simulink model "mvdc_vehicle_dynamics_control"  (R2018b)
settings: configuration reference "Active" (kept outside this file)
undefined symbols (not defined in the file): IC_TUMModeControl, tS
libraries: simulink x1
settings Model: DataDictionary=mvdc_vehicle_dynamics_control.sldd  Creator=wischnewski  LastModifiedBy=ga25xiw

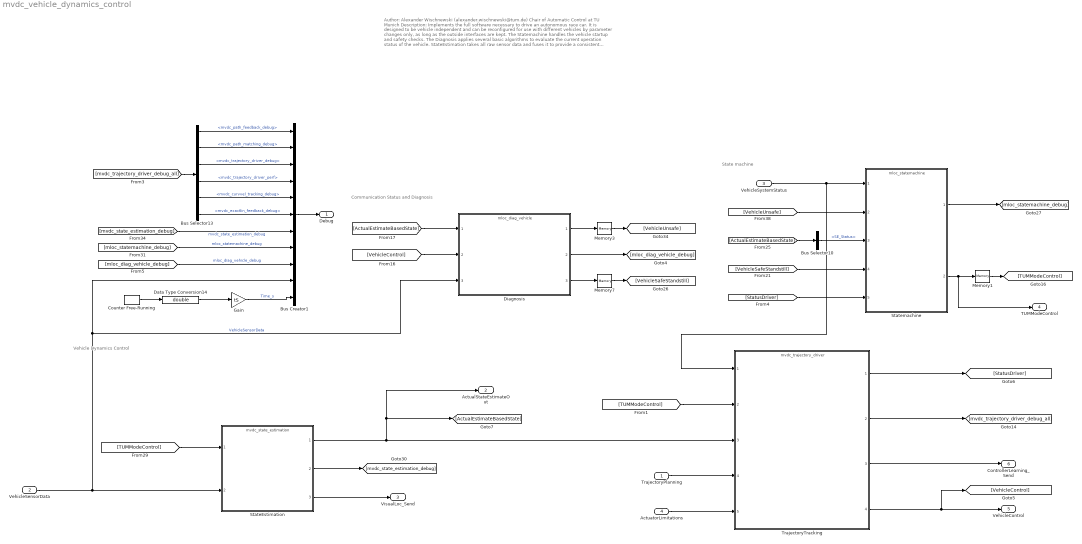
== system mvdc_vehicle_dynamics_control ==
  note: Communication Status and Diagnosis
  note: Vehicle Dynamics Control
  note: State machine
  note: Author: Alexander Wischnewski (alexander.wischnewski@tum.de)
      | Chair of Automatic Control at TU Munich
      |
      | Description: Implements the full software necessary to drive an autonomous race car. It is designed to be vehicle independent and
      | can be reconfigured for use with different vehicles by parameter changes only, as long as the outside interfaces are kept.
      |
      | The Statemachine handles the vehicle startup and safety checks.
      |
      | The Diagnosis applies several basic algorithms to evaluate the current operation status of the vehicle.
      |
      | StateEstimation takes all raw sensor data and fuses it to provide a consistent vehicle state estimate (position, velocity, etc.)
      |
      | The TrajectoryTracking fulfills the complete control tasks. It provides two options for controlling the vehicle:
      | 1) A lateral path PD-controller in combination with a curvature and velocity controller.
      | 2) An exact linearization based controller utilizing steady-state solutions of the lateral vehicle dynamics.
      |
      | Inputs:
      | TrajectoryPlanning Inputs from the trajectory planner
      | VehicleSensorData Raw sensor data for all vehicle sesnsors
      | VehicleSystemStatus Vehicle system status bits, e.g. sensor and actuator status
      | ActuatorLimitations Vehicle actuator limitations to be respected by the controller
      |
      | Outputs:
      | Debug debug bus which includes all component debug information
      | ActualStateEstimateOut Outputs currentvehicle state estimate
      | VisualLoc_Send Interface to LIDAR localization
      | TUMModeControl State machine interface to other algorithms
      | VehicleControl Vehicle control requests (steering and longitudinal force)
      | ControllerLearning_Send Interface to the controller learning algorithms
  TrajectoryPlanning : Inport  OutDataTypeStr=Bus: TrajectoryPlanning  BusOutputAsStruct=on
  VehicleSensorData : Inport  Port=2  OutDataTypeStr=Bus: VehicleSensorData  BusOutputAsStruct=on
  VehicleSystemStatus : Inport  Port=3  OutDataTypeStr=Bus: VehicleSystemStatus  BusOutputAsStruct=on
  ActuatorLimitations : Inport  Port=4  OutDataTypeStr=Bus: ActuatorLimitations  BusOutputAsStruct=on
  Bus Creator1 : BusCreator  Inputs=11
  Bus Selector10 : BusSelector  OutputSignals=SE_Status
  Bus Selector13 : BusSelector  OutputSignals=mvdc_path_feedback_debug,mvdc_path_matching_debug,mvdc_trajectory_driver_debug,mvdc_trajectory_driver_perf,mvdc_curvvel_tracking_debug,mvdc_exactlin_feedback_debug
  Counter Free-Running : simulink/Sources/Counter Free-Running  NumBits=32  tsamp=tS
  Data Type Conversion14 : DataTypeConversion  OutDataTypeStr=double
  Diagnosis : ModelReference  ModelNameDialog=mloc_diag_vehicle.slx  SimulationMode=Normal  ModelReferenceVersion=1.75
  Gain : Gain  Gain=tS
  Memory1 : Memory  InitialCondition=IC_TUMModeControl
  Memory3 : Memory  InitialCondition=uint16(0)
  Memory7 : Memory  InitialCondition=uint16(0)
  StateEstimation : ModelReference  ModelNameDialog=mvdc_state_estimation  SimulationMode=Normal  ModelReferenceVersion=1.950
  Statemachine : ModelReference  ModelNameDialog=mloc_statemachine.slx  SimulationMode=Normal  ModelReferenceVersion=1.463
  TrajectoryTracking : ModelReference  ModelNameDialog=mvdc_trajectory_driver.slx  SimulationMode=Normal  ModelReferenceVersion=1.798
  Debug : Outport  OutDataTypeStr=Bus: mvdc_vehicle_dynamics_control_debug  BusOutputAsStruct=on
  ActualStateEstimateOut : Outport  Port=2  OutDataTypeStr=Bus: VehicleDynamicState  BusOutputAsStruct=on
  VisualLoc_Send : Outport  Port=3  OutDataTypeStr=Bus: VisualLoc_Send  BusOutputAsStruct=on
  TUMModeControl : Outport  Port=4  OutDataTypeStr=Bus: TUMModeControl  BusOutputAsStruct=on
  VehicleControl : Outport  Port=5  OutDataTypeStr=Bus: VehicleControl  BusOutputAsStruct=on
  ControllerLearning_Send : Outport  Port=6  OutDataTypeStr=Bus: ControllerLearning_Send  BusOutputAsStruct=on
  wires:
  Bus Creator1/1 -> Debug/1
  StateEstimation/2 -> [mvdc_state_estimation_debug]
  [mvdc_state_estimation_debug] -> Bus Creator1/7  "mvdc_state_estimation_debug"
  [ActualEstimateBasedState] -> Diagnosis/1
  Memory3/1 -> [VehicleUnsafe]
  [mloc_diag_vehicle_debug] -> Bus Creator1/9  "mloc_diag_vehicle_debug"
  [VehicleControl] -> Diagnosis/2
  Memory7/1 -> [VehicleSafeStandstill]
  Diagnosis/3 -> Memory7/1
  Statemachine/2 -> TUMModeControl/1, Memory1/1
  Memory1/1 -> [TUMModeControl]
  Counter Free-Running/1 -> Data Type Conversion14/1
  Gain/1 -> Bus Creator1/11  "Time_s"
  Data Type Conversion14/1 -> Gain/1
  VehicleSensorData/1 -> Diagnosis/3, Bus Creator1/10, StateEstimation/2  "VehicleSensorData"
  [ActualEstimateBasedState] -> Bus Selector10/1
  StateEstimation/3 -> VisualLoc_Send/1
  Diagnosis/1 -> Memory3/1
  Diagnosis/2 -> [mloc_diag_vehicle_debug]
  TrajectoryPlanning/1 -> TrajectoryTracking/4
  Statemachine/1 -> [mloc_statemachine_debug]
  VehicleSystemStatus/1 -> TrajectoryTracking/1, Statemachine/1
  Bus Selector10/1 -> Statemachine/3  "<SE_Status>"
  [VehicleUnsafe] -> Statemachine/2
  [VehicleSafeStandstill] -> Statemachine/4
  [StatusDriver] -> Statemachine/5
  TrajectoryTracking/1 -> [StatusDriver]
  StateEstimation/1 -> ActualStateEstimateOut/1, [ActualEstimateBasedState], TrajectoryTracking/3
  [mvdc_trajectory_driver_debug_all] -> Bus Selector13/1
  Bus Selector13/3 -> Bus Creator1/3  "<mvdc_trajectory_driver_debug>"
  Bus Selector13/4 -> Bus Creator1/4  "<mvdc_trajectory_driver_perf>"
  Bus Selector13/2 -> Bus Creator1/2  "<mvdc_path_matching_debug>"
  Bus Selector13/1 -> Bus Creator1/1  "<mvdc_path_feedback_debug>"
  [mloc_statemachine_debug] -> Bus Creator1/8  "mloc_statemachine_debug"
  TrajectoryTracking/3 -> ControllerLearning_Send/1
  ActuatorLimitations/1 -> TrajectoryTracking/5
  TrajectoryTracking/2 -> [mvdc_trajectory_driver_debug_all]
  TrajectoryTracking/4 -> VehicleControl/1, [VehicleControl]
  Bus Selector13/5 -> Bus Creator1/5  "<mvdc_curvvel_tracking_debug>"
  Bus Selector13/6 -> Bus Creator1/6  "<mvdc_exactlin_feedback_debug>"
  [TUMModeControl] -> StateEstimation/1
  [TUMModeControl] -> TrajectoryTracking/2
